simulink model "no1_proportional_controller"  (R2025a)
settings: Solver=VariableStepAuto  StartTime=0.0  StopTime=50  RelTol=1e-3
settings Model: Creator=ayeo  LastModifiedBy=ayeo

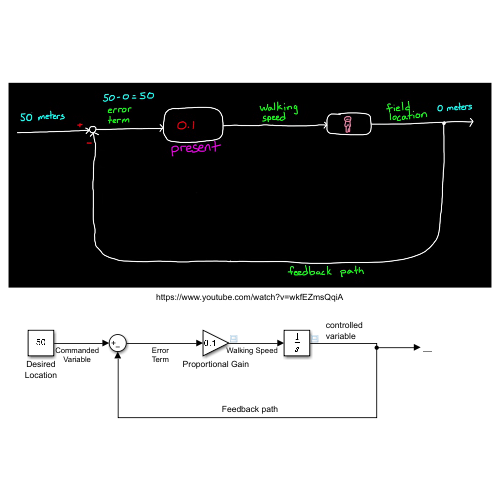
[thumbnail: Simulink's stored preview of the top-level diagram]
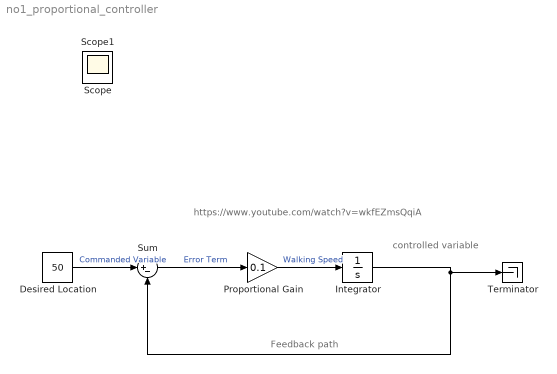
== system no1_proportional_controller ==
  note: https://www.youtube.com/watch?v=wkfEZmsQqiA
  note: controlled
      | variable
  note: Feedback path
  Desired Location : Constant  Value=50
  Integrator : Integrator
  Proportional Gain : Gain  Gain=0.1
  Sum : Sum  Inputs=|+-
  Terminator : Terminator
  Scope : Scope
      settings: ActiveDisplayYMinimum=-6.2078878305767491  ActiveDisplayYMaximum=55.870990475190759
  Scope1 : Scope
      settings: ActiveDisplayYMinimum=-0.58709904751907571  ActiveDisplayYMaximum=5.6207887830576748
  wires:
  Desired Location/1 -> Sum/1  "Commanded Variable"
  Sum/1 -> Proportional Gain/1  "Error Term"
  Proportional Gain/1 -> Integrator/1  "Walking Speed"
  Integrator/1 -> Sum/2, Terminator/1
